simulink model "Joystick_test"  (R2012b)
settings: Solver=ode45  StartTime=0.0  StopTime=inf  RelTol=1e-3
libraries: vrlib x1, rtwinlib x1
settings Model: Creator=David  LastModifiedBy=David

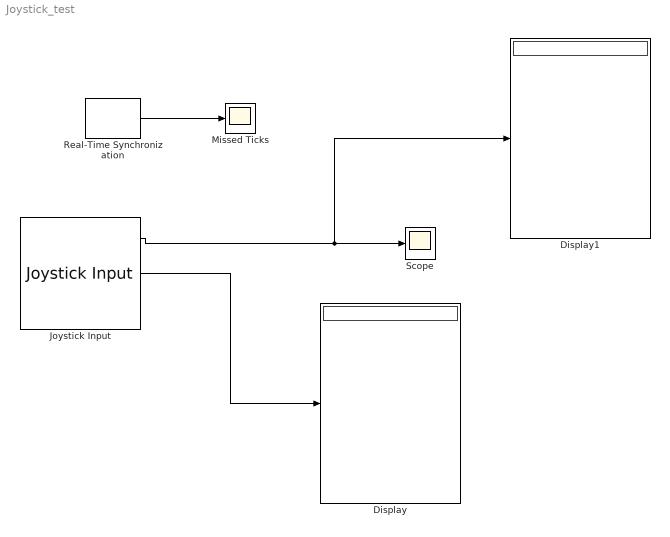
== system Joystick_test ==
  Display : Display
  Display1 : Display
  Joystick Input : vrlib/Joystick Input  joyid=1  adjustports=on  forcefeed=off
  Missed Ticks : Scope
      settings: TickLabels=on  TimeRange=20  YMin=0  YMax=30
  Real-Time Synchronization : rtwinlib/Real-Time Synchronization  SampleTime=0.001  MaxMissedTicks=100000  ShowMissedTicks=on  YieldWhenWaiting=on
  Scope : Scope
  wires:
  Joystick Input/1 -> Display1/1, Scope/1
  Real-Time Synchronization/1 -> Missed Ticks/1
  Joystick Input/2 -> Display/1
